simulink model "three_phase_rect"  (R2016a)
settings: Solver=ode4  StartTime=0.0  StopTime=2  FixedStep=1e-5  RelTol=1e-3
libraries: powerlib x10, powerlib_meascontrol x7
settings Model: Creator=ugurm  LastModifiedBy=mesutto
settings DataIOCC: LimitDataPoints=on  SaveFormat=Array
settings DebuggingCC: UnderspecifiedInitializationDetection=Classic  MergeDetectMultiDrivingBlocksExec=none  SolverPrmCheckMsg=warning  StateNameClashWarn=warning
settings HardwareCC: ProdBitPerPointer=32  ProdLargestAtomicFloat=None  ProdIntDivRoundTo=Undefined  ProdEndianess=Unspecified  ProdWordSize=32  ProdHWDeviceType=32-bit Generic
settings ModelReferenceCC: PropagateSignalLabelsOutOfModel=off
settings ConfigComp: CovModelRefEnable=Off

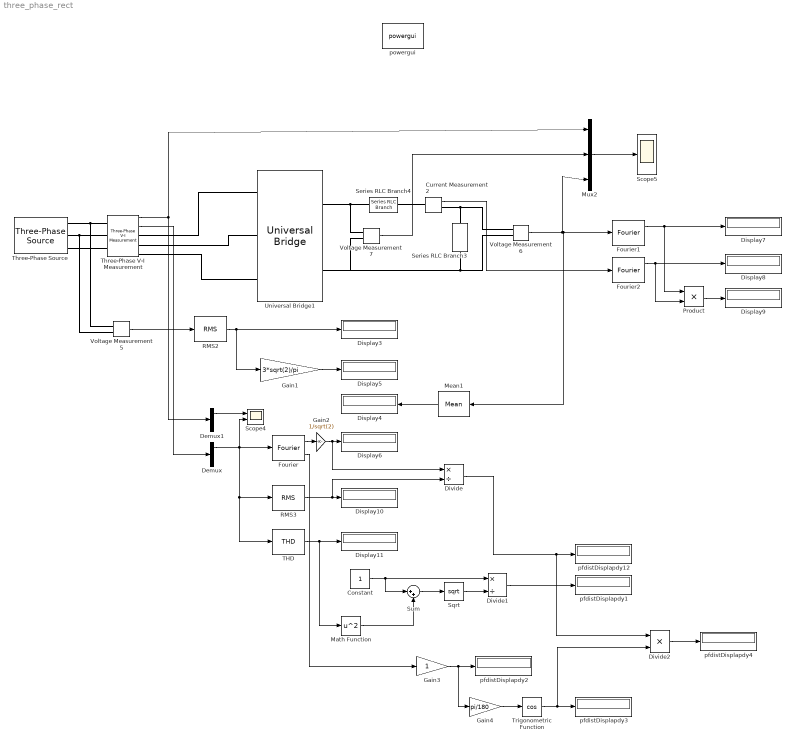
== system three_phase_rect ==
  Constant : Constant
  Current Measurement2 : powerlib/Measurements/Current Measurement  PhasorSimulation=off  OutputType=Complex  PSBequivalent=0
  Demux : Demux  Outputs=3
  Demux1 : Demux  Outputs=3
  Display{3..11} (9 alike) : Display
  Divide : Product  Inputs=*/
  Divide1 : Product  Inputs=*/
  Divide2 : Product  Inputs=**
  Fourier : powerlib_meascontrol/Measurements/Fourier  Freq=50  n=1  InInit=[0, 0]  Ts=0
  Fourier1 : powerlib_meascontrol/Measurements/Fourier  Freq=50  n=0  InInit=[0, 0]  Ts=0
  Fourier2 : powerlib_meascontrol/Measurements/Fourier  Freq=50  n=0  InInit=[0, 0]  Ts=0
  Gain1 : Gain  Gain=3*sqrt(2)/pi
  Gain2 : Gain  Gain=1/sqrt(2)
  Gain3 : Gain
  Gain4 : Gain  Gain=pi/180
  Math Function : Math  Operator=square  SaturateOnIntegerOverflow=on
  Mean1 : powerlib_meascontrol/Measurements/Mean  Freq=50  Vinit=0  Ts=0
  Mux2 : Mux  Inputs=3
  Product : Product
  RMS2 : powerlib_meascontrol/Measurements/RMS  TrueRMS=on  Freq=50  RMSInit=0  Ts=0
  RMS3 : powerlib_meascontrol/Measurements/RMS  TrueRMS=on  Freq=50  RMSInit=0  Ts=0
  Scope4 : Scope  NumInputPorts=2
  Scope5 : Scope
  Series RLC Branch3 : powerlib/Elements/Series RLC Branch  LConnTagsString=__new0  RConnTagsString=__new0  BranchType=R  Resistance=5.4  Inductance=1/(2*pi*50)  SetiL0=off  InitialCurrent=0  Capacitance=1e-6  Setx0=off  InitialVoltage=0  Measurements=None
  Series RLC Branch4 : powerlib/Elements/Series RLC Branch  LConnTagsString=__new0  RConnTagsString=__new0  BranchType=L  Resistance=2  Inductance=100/(2*pi*50)  SetiL0=off  InitialCurrent=0  Capacitance=1e-6  Setx0=off  InitialVoltage=0  Measurements=None
  Sqrt : Sqrt  SaturateOnIntegerOverflow=on
  Sum : Sum  Inputs=|++
  THD : powerlib_meascontrol/Measurements/THD  Freq=50  Ts=0
  Three-Phase V-I Measurement : powerlib/Measurements/Three-Phase V-I Measurement  VoltageMeasurement=phase-to-ground  SetLabelV=off  LabelV=Vabc  Vpu=off  VpuLL=off  CurrentMeasurement=yes  SetLabelI=off  LabelI=Iabc  Ipu=off  Pbase=100e6  Vbase=500e3  OutputType=Complex  PhasorSimulation=off  PSBequivalent=0
  Three-Phase Source : powerlib/Electrical Sources/Three-Phase Source  InternalConnection=Yg  VoltagePhases=off  Voltage=400  PhaseAngle=0  Voltage_phases=[25e3 25e3 25e3]/sqrt(3)  PhaseAngles_phases=[0 -120 +120]  Frequency=50  NonIdealSource=off  SpecifyImpedance=off  Resistance=0.8929  Inductance=16.58e-3  ShortCircuitLevel=100e6  BaseVoltage=25e3  XRratio=7  BusType=swing  Pref=10e3  Qref=0  Prefabc=[10e3, 10e3, 10e3]  Qrefabc=[0, 0, 0]  Qmin=-inf  Qmax=inf
  Trigonometric Function : Trigonometry  Operator=cos
  Universal Bridge1 : powerlib/Power Electronics/Universal Bridge  Arms=3  SnubberResistance=1e5  SnubberCapacitance=inf  Device=Diodes  Ron=1e-3  Lon=0  ForwardVoltages="[  0  0  ]"  ForwardVoltage=0  GTOparameters=[ 10e-6 , 20e-6 ]  IGBTparameters=[ 1e-6 , 2e-6 ]  Measurements=None  Measurements_2=None  converterType=Rectifier
  Voltage Measurement5 : powerlib/Measurements/Voltage Measurement  PhasorSimulation=off  OutputType=Complex  PSBequivalent=0
  Voltage Measurement6 : powerlib/Measurements/Voltage Measurement  PhasorSimulation=off  OutputType=Complex  PSBequivalent=0
  Voltage Measurement7 : powerlib/Measurements/Voltage Measurement  PhasorSimulation=off  OutputType=Complex  PSBequivalent=0
  pfdistDisplapdy{1..4,12} (5 alike) : Display
  powergui : powerlib/powergui  Priority=1  SimulationMode=Discrete  SolverType=Tustin/Backward Euler (TBE)  SampleTime=1e-5  frequency=60  SPID=off  DisableSnubberDevices=off  DisableRonSwitches=off  DisableVfSwitches=off  SwTol=0  DisplayEquations=off  Interpol=off  ExternalGateDelay=off  methode=off  Ts=10  FunctionMessages=off  echomessages=off  HookPort=off  EnableUseOfTLC=off  x0status=blocks  frequencyindice=50  Pbase=100e6  ErrMax=1e-4  Iterations=50  UnitsV=kV  UnitsW=MW  buscounter=0  RestoreLinks=warning  ResistiveCurrentMeasurement=off  Frange=[0:2:500]  Ylog=off  Xlog=on  ShowGrid=off  save=off  variable=ZData  structure=vdc  ZoomFFT=off  StartTime=0.2  cycles=20  DisplayStyle=5  fundamental=50  FreqAxis=off  MaxFrequency=2000  frequencyindicesteady=1  RmsSteady=1  display=off
  wires:
  Voltage Measurement6/1 -> Mux2/3, Mean1/1, Fourier1/1
  RMS2/1 -> Gain1/1, Display3/1
  Mean1/1 -> Display4/1
  Gain1/1 -> Display5/1
  Three-Phase V-I Measurement/1 -> Demux1/1, Mux2/1
  Voltage Measurement7/1 -> Mux2/2
  Mux2/1 -> Scope5/1
  Voltage Measurement5/1 -> RMS2/1
  Three-Phase V-I Measurement/2 -> Demux/1
  Demux/1 -> THD/1, RMS3/1, Scope4/2, Fourier/1
  Fourier/1 -> Gain2/1
  Current Measurement2/1 -> Fourier2/1
  Fourier1/1 -> Product/1, Display7/1
  Fourier2/1 -> Product/2, Display8/1
  Product/1 -> Display9/1
  Demux1/1 -> Scope4/1
  RMS3/1 -> Divide/2, Display10/1
  Gain2/1 -> Divide/1, Display6/1
  THD/1 -> Math Function/1, Display11/1
  Divide/1 -> Divide2/1, pfdistDisplapdy12/1
  Constant/1 -> Sum/1, Divide1/1
  Sqrt/1 -> Divide1/2
  Math Function/1 -> Sum/2
  Sum/1 -> Sqrt/1
  Divide1/1 -> pfdistDisplapdy1/1
  Fourier/2 -> Gain3/1
  Gain3/1 -> Gain4/1, pfdistDisplapdy2/1
  Trigonometric Function/1 -> Divide2/2, pfdistDisplapdy3/1
  Divide2/1 -> pfdistDisplapdy4/1
  Gain4/1 -> Trigonometric Function/1
  connections:
  Voltage Measurement6/LConn1 -- Current Measurement2/RConn1 -- Series RLC Branch3/LConn1
  Voltage Measurement6/LConn2 -- Voltage Measurement7/LConn2 -- Universal Bridge1/RConn2 -- Series RLC Branch3/RConn1
  Series RLC Branch4/RConn1 -- Universal Bridge1/RConn1 -- Voltage Measurement7/LConn1
  Three-Phase V-I Measurement/LConn1 -- Voltage Measurement5/LConn1 -- Three-Phase Source/RConn1
  Three-Phase Source/RConn2 -- Voltage Measurement5/LConn2 -- Three-Phase V-I Measurement/LConn2
  Three-Phase Source/RConn3 -- Three-Phase V-I Measurement/LConn3
  Three-Phase V-I Measurement/RConn1 -- Universal Bridge1/LConn1
  Three-Phase V-I Measurement/RConn2 -- Universal Bridge1/LConn2
  Three-Phase V-I Measurement/RConn3 -- Universal Bridge1/LConn3
  Current Measurement2/LConn1 -- Series RLC Branch4/LConn1
